simulink model "panelMotor_control_power_2018"  (R2018a)
settings: Solver=VariableStepAuto  StartTime=0.0  StopTime=150*3600  RelTol=1e-3
values from neighbouring files (symbols this model uses):
  A = w*l    (= 1.456)    [panelMotorParams.m]
  beta = pi/4    (= 0.785398163397)    [panelMotorParams.m]
  J = m/12*(l^2*cos(beta)^2+d^2*sin(beta)^2+w^2)    [panelMotorParams.m]
  Kd = 5    [panelMotorParams.m]
  Kf = 0.07    [panelMotorParams.m]
  Kg = 2000    [panelMotorParams.m]
  Kt = 0.07    [panelMotorParams.m]
  L = 1e-5    (= 1e-05)    [panelMotorParams.m]
  R = 10    [panelMotorParams.m]
libraries: simulink x1
settings Model: Creator=goku-ubuntu  LastModifiedBy=goku-ubuntu
settings DataIOCC: ExternalInput=[sunTime, sunPosition, sunElevation]  LoadExternalInput=on

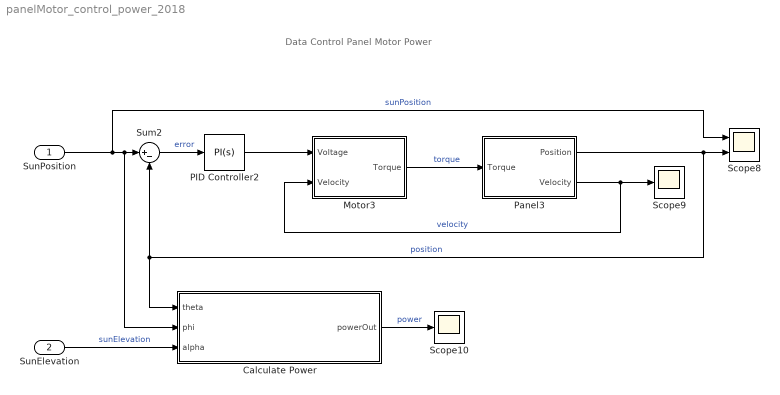
== system panelMotor_control_power_2018 ==
  note: Data Control Panel Motor Power
  SunPosition : Inport
  SunElevation : Inport  Port=2
  Calculate Power : MATLAB Function  TreatAsAtomicUnit=on
  Motor3 : Subsystem
  PID Controller2 : simulink/Continuous/PID Controller  Controller=PI  TimeDomain=Continuous-time  SampleTime=-1  IntegratorMethod=Forward Euler  FilterMethod=Forward Euler  Form=Parallel  UseFilter=on  ControllerParametersSource=internal  P=240  I=180  D=0  N=100  InitialConditionSource=internal  InitialConditionForIntegrator=0  InitialConditionForFilter=0  ExternalReset=none  LimitOutput=off  UpperSaturationLimit=inf  LowerSaturationLimit=-inf  LinearizeAsGain=on  AntiWindupMode=none  Kb=1  TrackingMode=off  Kt=1  PParamMin=[]  PParamMax=[]  IParamMin=[]  IParamMax=[]  DParamMin=[]  DParamMax=[]  NParamMin=[]  NParamMax=[]  KbParamMin=[]  KbParamMax=[]  KtParamMin=[]  KtParamMax=[]  POutMin=[]  POutMax=[]  IOutMin=[]  IOutMax=[]  DOutMin=[]  DOutMax=[]  NOutMin=[]  NOutMax=[]  KbOutMin=[]  KbOutMax=[]  KtOutMin=[]  KtOutMax=[]  IntegratorOutMin=[]  IntegratorOutMax=[]  FilterOutMin=[]  FilterOutMax=[]  SumOutMin=[]  SumOutMax=[]  SumI1OutMin=[]  SumI1OutMax=[]  SumI2OutMin=[]  SumI2OutMax=[]  SumI3OutMin=[]  SumI3OutMax=[]  SumDOutMin=[]  SumDOutMax=[]  SaturationOutMin=[]  SaturationOutMax=[]  IntegratorContinuousStateAttributes=''  IntegratorStateMustResolveToSignalObject=off  IntegratorRTWStateStorageClass=Auto  FilterContinuousStateAttributes=''  FilterStateMustResolveToSignalObject=off  FilterRTWStateStorageClass=Auto  DifferentiatorICPrevScaledInput=0  DifferentiatorOutMin=[]  DifferentiatorOutMax=[]  FilterDiffOutCoefMin=[]  FilterDiffOutCoefMax=[]  SumDenOutMin=[]  SumDenOutMax=[]  SumNumOutMin=[]  SumNumOutMax=[]  ReciprocalOutMin=[]  ReciprocalOutMax=[]  DivideOutMin=[]  DivideOutMax=[]  TunerSelectOption=Transfer Function Based (PID Tuner App)
  Panel3 : Subsystem
  Scope10 : Scope
  Scope8 : Scope  NumInputPorts=2
  Scope9 : Scope
  Sum2 : Sum  Inputs=|+-
  wires:
  SunElevation/1 -> Calculate Power/3(alpha)  "sunElevation"
  Panel3/2(Velocity) -> Motor3/2(Velocity), Scope9/1  "velocity"
  PID Controller2/1 -> Motor3/1(Voltage)
  Sum2/1 -> PID Controller2/1  "error"
  Calculate Power/1(powerOut) -> Scope10/1  "power"
  Motor3/1(Torque) -> Panel3/1(Torque)  "torque"
  SunPosition/1 -> Calculate Power/2(phi), Sum2/1, Scope8/1  "sunPosition"
  Panel3/1(Position) -> Scope8/2, Sum2/2, Calculate Power/1(theta)  "position"

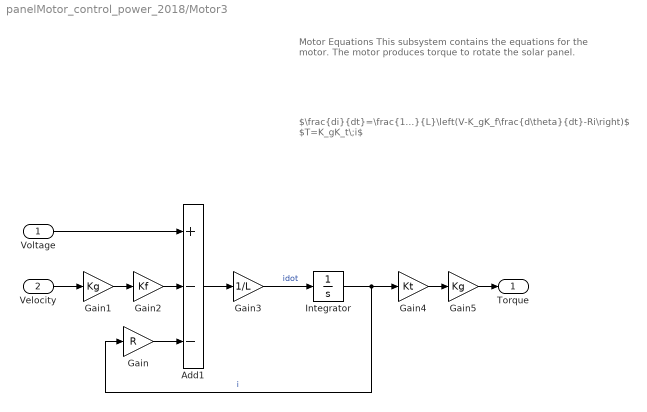
== system panelMotor_control_power_2018/Motor3 ==
  note: $\frac{di}{dt}=\frac{1}{L}\left(V-K_gK_f\frac{d\theta}{dt}-Ri\right)$
      | $T=K_gK_t\;i$
  note: Motor Equations
      |
      | This subsystem contains the equations for the motor. The motor produces torque to rotate the solar panel.
  Voltage : Inport
  Velocity : Inport  Port=2
  Add1 : Sum  Inputs=+--
  Gain : Gain  Gain=R
  Gain1 : Gain  Gain=Kg
  Gain2 : Gain  Gain=Kf
  Gain3 : Gain  Gain=1/L
  Gain4 : Gain  Gain=Kt
  Gain5 : Gain  Gain=Kg
  Integrator : Integrator
  Torque : Outport  VectorParamsAs1DForOutWhenUnconnected=on
  wires:
  Voltage/1 -> Add1/1
  Gain2/1 -> Add1/2
  Gain3/1 -> Integrator/1  "idot"
  Gain/1 -> Add1/3
  Integrator/1 -> Gain4/1, Gain/1  "i"
  Add1/1 -> Gain3/1
  Velocity/1 -> Gain1/1
  Gain4/1 -> Gain5/1
  Gain1/1 -> Gain2/1
  Gain5/1 -> Torque/1

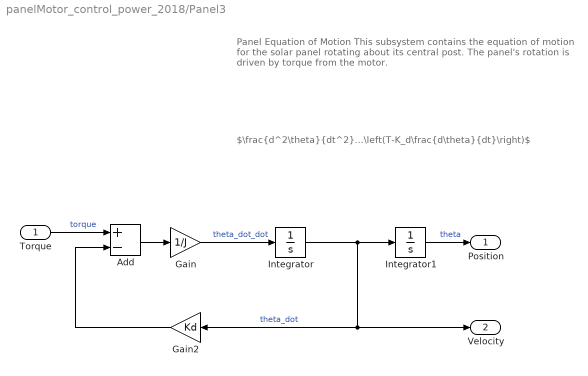
== system panelMotor_control_power_2018/Panel3 ==
  note: $\frac{d^2\theta}{dt^2}=\frac{1}{J}\left(T-K_d\frac{d\theta}{dt}\right)$
  note: Panel Equation of Motion
      |
      | This subsystem contains the equation of motion for the solar panel rotating about its central post. The panel's rotation is driven by torque from the motor.
  Torque : Inport
  Add : Sum  Inputs=+-
  Gain : Gain  Gain=1/J
  Gain2 : Gain  Gain=Kd
  Integrator : Integrator
  Integrator1 : Integrator
  Position : Outport  VectorParamsAs1DForOutWhenUnconnected=on
  Velocity : Outport  Port=2  VectorParamsAs1DForOutWhenUnconnected=on
  wires:
  Torque/1 -> Add/1  "torque"
  Add/1 -> Gain/1
  Integrator/1 -> Integrator1/1, Velocity/1, Gain2/1  "theta_dot"
  Gain2/1 -> Add/2
  Gain/1 -> Integrator/1  "theta_dot_dot"
  Integrator1/1 -> Position/1  "theta"

== matlab function panelMotor_control_power_2018/Calculate Power ==
  data: theta input; phi input; alpha input; powerOut output; A parameter; beta parameter
function powerOut = CalculatePower(theta, phi, alpha, A, beta)

% Calculate dot product of the incident sun and panel normal vectors
dot_prod = sin(beta)*sin(pi/2-alpha)*cos(theta-phi) ...
    + cos(beta)*cos(pi/2-alpha);

% Calculate the direct power
powerOut = 1.353*0.7.^(sin(alpha).^-0.678)*dot_prod*A*0.195*1000; % W

% Replace negative power values with zero (sun is behind the panel)
powerOut = max(powerOut,0);
